simulink model "electromagnetic_piston"  (R2024a)
settings: Solver=VariableStepAuto  StartTime=0.0  StopTime=10.0  RelTol=1e-3
undefined symbols (not defined in the file): alpha0, beta1, beta2, c, C_T, h, k1, k3, L0, m, R, T0, T_env, x_eq
settings Model: Creator=Bocchio  LastModifiedBy=Bocchio

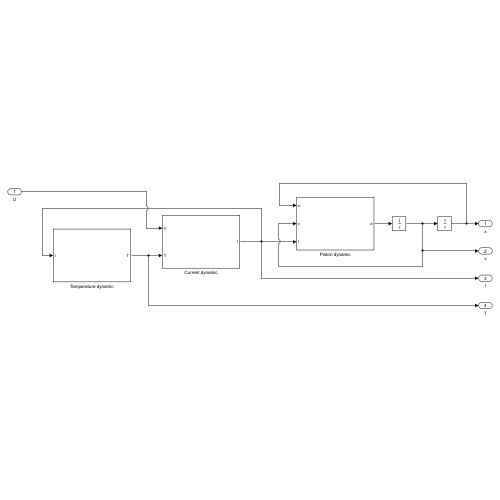
[thumbnail: Simulink's stored preview of the top-level diagram]
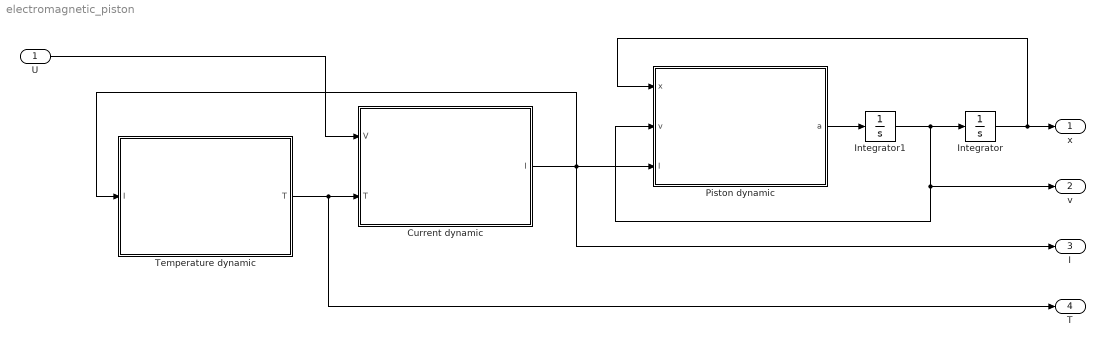
== system electromagnetic_piston ==
  U : Inport
  Current dynamic : Subsystem
  Integrator : Integrator  InitialCondition=x_eq(1)
  Integrator1 : Integrator
  Piston dynamic : Subsystem
  Temperature dynamic : Subsystem
  x : Outport
  v : Outport  Port=2
  I : Outport  Port=3
  T : Outport  Port=4
  wires:
  Integrator/1 -> Piston dynamic/1(x), x/1
  Integrator1/1 -> Integrator/1, v/1, Piston dynamic/2(v)
  Current dynamic/1(I) -> I/1, Temperature dynamic/1(I), Piston dynamic/3(I)
  U/1 -> Current dynamic/1(V)
  Piston dynamic/1(a) -> Integrator1/1
  Temperature dynamic/1(T) -> T/1, Current dynamic/2(T)

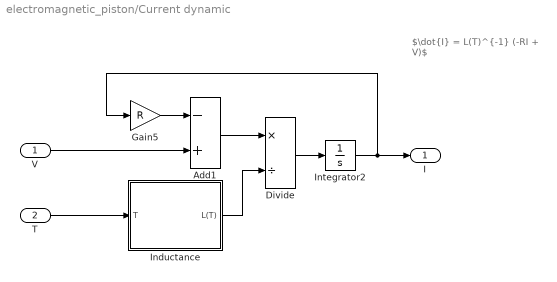
== system electromagnetic_piston/Current dynamic ==
  note: $\dot{I} = L(T)^{-1} (-RI + V)$
  V : Inport
  T : Inport  Port=2
  Add1 : Sum  Inputs=-+
  Divide : Product  Inputs=*/
  Gain5 : Gain  Gain=R
  Inductance : Subsystem
  Integrator2 : Integrator  InitialCondition=x_eq(3)
  I : Outport
  wires:
  Integrator2/1 -> I/1, Gain5/1
  Gain5/1 -> Add1/1
  T/1 -> Inductance/1(T)
  Add1/1 -> Divide/1
  Divide/1 -> Integrator2/1
  Inductance/1(L(T)) -> Divide/2
  V/1 -> Add1/2

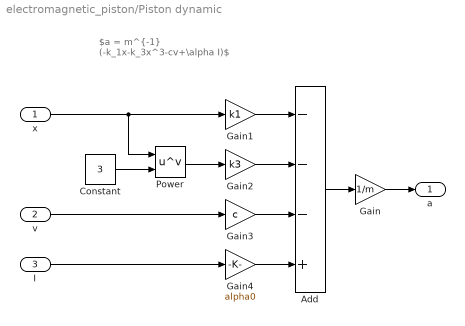
== system electromagnetic_piston/Piston dynamic ==
  note: $a = m^{-1} (-k_1x-k_3x^3-cv+\alpha I)$
  x : Inport
  v : Inport  Port=2
  I : Inport  Port=3
  Add : Sum  Inputs=---+
  Constant : Constant  Value=3
  Gain : Gain  Gain=1/m
  Gain1 : Gain  Gain=k1
  Gain2 : Gain  Gain=k3
  Gain3 : Gain  Gain=c
  Gain4 : Gain  Gain=alpha0
  Power : Math  Operator=pow
  a : Outport
  wires:
  x/1 -> Gain1/1, Power/1
  v/1 -> Gain3/1
  Gain2/1 -> Add/2
  Power/1 -> Gain2/1
  Add/1 -> Gain/1
  Gain4/1 -> Add/4
  Gain1/1 -> Add/1
  Gain3/1 -> Add/3
  I/1 -> Gain4/1
  Constant/1 -> Power/2
  Gain/1 -> a/1

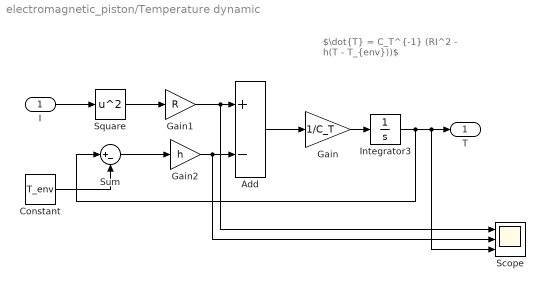
== system electromagnetic_piston/Temperature dynamic ==
  note: $\dot{T} = C_T^{-1} (RI^2 - h(T - T_{env}))$
  I : Inport
  Add : Sum  Inputs=+-
  Constant : Constant  Value=T_env
  Gain : Gain  Gain=1/C_T
  Gain1 : Gain  Gain=R
  Gain2 : Gain  Gain=h
  Integrator3 : Integrator  InitialCondition=x_eq(4)
  Scope : Scope  NumInputPorts=3
  Square : Math  Operator=square
  Sum : Sum  Inputs=|+-
  T : Outport
  wires:
  I/1 -> Square/1
  Integrator3/1 -> Sum/1, Scope/3, T/1
  Gain/1 -> Integrator3/1
  Square/1 -> Gain1/1
  Add/1 -> Gain/1
  Gain1/1 -> Scope/1, Add/1
  Gain2/1 -> Scope/2, Add/2
  Sum/1 -> Gain2/1
  Constant/1 -> Sum/2

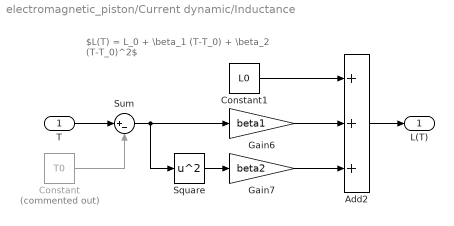
== system electromagnetic_piston/Current dynamic/Inductance ==
  note: $L(T) = L_0 + \beta_1 (T-T_0) + \beta_2 (T-T_0)^2$
  T : Inport
  Add2 : Sum  Inputs=+++
  Constant : Constant  Commented=on  Value=T0
  Constant1 : Constant  Value=L0
  Gain6 : Gain  Gain=beta1
  Gain7 : Gain  Gain=beta2
  Square : Math  Operator=square
  Sum : Sum  Inputs=|+-
  L(T) : Outport
  wires:
  Square/1 -> Gain7/1
  Gain6/1 -> Add2/2
  Gain7/1 -> Add2/3
  Constant1/1 -> Add2/1
  Add2/1 -> L(T)/1
  Constant/1 -> Sum/2
  T/1 -> Sum/1
  Sum/1 -> Gain6/1, Square/1
